simulink model "systemmodel"  (R2013b)
settings: Solver=ode45  StartTime=0.0  StopTime=10.0  RelTol=1e-3
values from neighbouring files (symbols this model uses):
  J_m1 = mean(J_1)    [identifier.m]
  J_m2 = mean(J_2)    [identifier.m]
  K_m1 = mean(k_1)    [identifier.m]
  K_m2 = mean(k_2)    [identifier.m]
undefined symbols (not defined in the file or in its folder): L_m1, L_m2
settings Model: Creator=torbal  LastModifiedBy=torbal

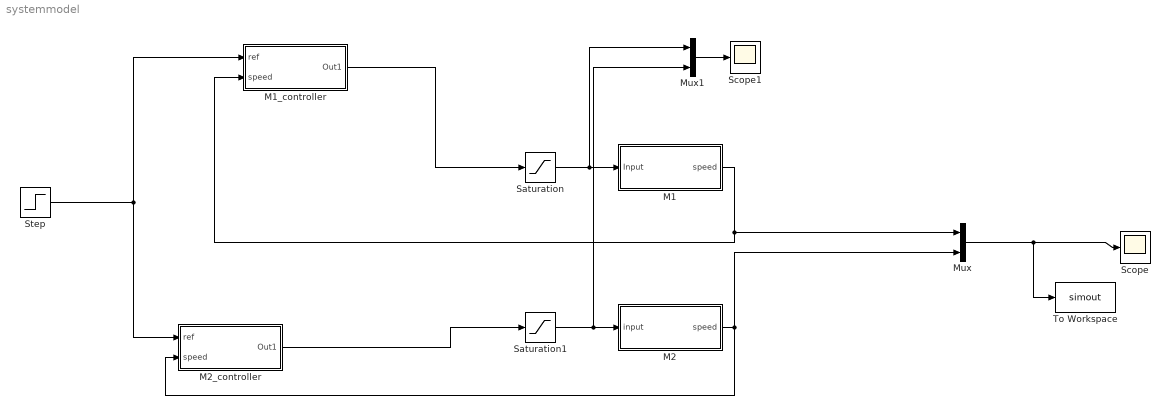
== system systemmodel ==
  M1 : Subsystem
  M1_controller : Subsystem
  M2 : Subsystem
  M2_controller : Subsystem
  Mux : Mux  Inputs=2
  Mux1 : Mux  Inputs=2
  Saturation : Saturate  UpperLimit=12  LowerLimit=-12
  Saturation1 : Saturate  UpperLimit=12  LowerLimit=-12
  Scope : Scope
      settings: TimeRange=10  YMin=0  YMax=60
  Scope1 : Scope
  Step : Step  After=50  SampleTime=0
  To Workspace : ToWorkspace  VariableName=simout  SampleTime=-1  SaveFormat=Timeseries
  wires:
  M2/1(speed) -> M2_controller/2(speed), Mux/2
  M1/1(speed) -> M1_controller/2(speed), Mux/1
  Mux/1 -> To Workspace/1, Scope/1
  M2_controller/1(Out1) -> Saturation1/1
  Saturation1/1 -> Mux1/2, M2/1(input)
  Saturation/1 -> Mux1/1, M1/1(Input)
  Mux1/1 -> Scope1/1
  Step/1 -> M1_controller/1("ref "), M2_controller/1("ref ")
  M1_controller/1(Out1) -> Saturation/1

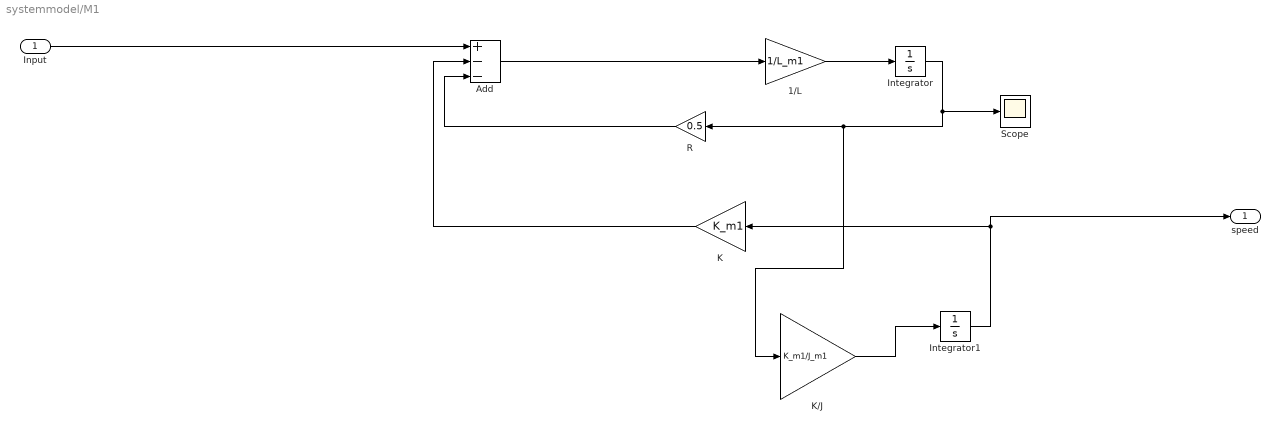
== system systemmodel/M1 ==
  Input : Inport
  1/L : Gain  Gain=1/L_m1
  Add : Sum  Inputs=+--
  Integrator : Integrator
  Integrator1 : Integrator
  K : Gain  Gain=K_m1
  K/J : Gain  Gain=K_m1/J_m1
  R : Gain  Gain=0.5
  Scope : Scope
      settings: SaveName=ScopeData2
  speed : Outport
  wires:
  1/L/1 -> Integrator/1
  Add/1 -> 1/L/1
  Input/1 -> Add/1
  K/J/1 -> Integrator1/1
  Integrator1/1 -> speed/1, K/1
  K/1 -> Add/2
  R/1 -> Add/3
  Integrator/1 -> K/J/1, R/1, Scope/1

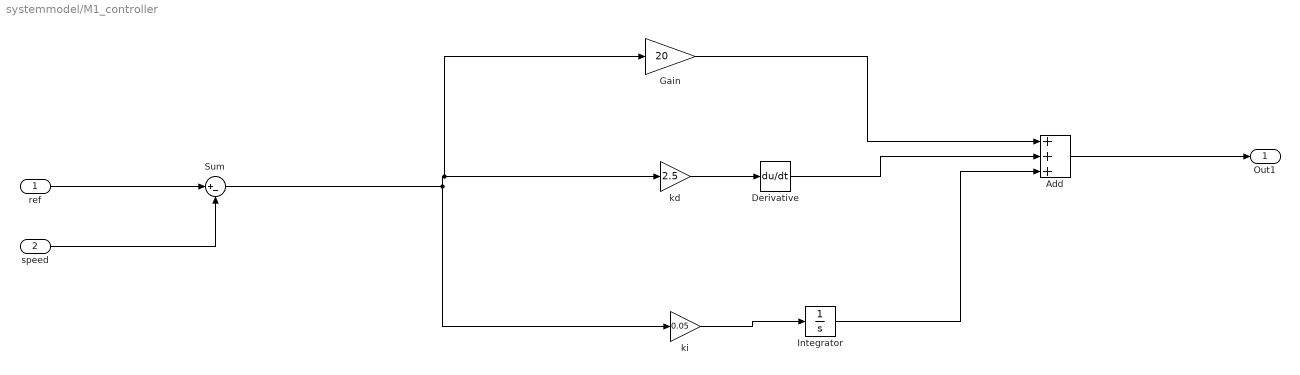
== system systemmodel/M1_controller ==
  "ref " : Inport
  speed : Inport  Port=2
  Add : Sum  Inputs=+++
  Derivative : Derivative
  Gain : Gain  Gain=20
  Integrator : Integrator
  Sum : Sum  Inputs=|+-
  "kd " : Gain  Gain=2.5
  ki : Gain  Gain=0.05
  Out1 : Outport
  wires:
  Gain/1 -> Add/1
  Add/1 -> Out1/1
  "ref "/1 -> Sum/1
  speed/1 -> Sum/2
  Sum/1 -> Gain/1, "kd "/1, ki/1
  "kd "/1 -> Derivative/1
  Derivative/1 -> Add/2
  ki/1 -> Integrator/1
  Integrator/1 -> Add/3

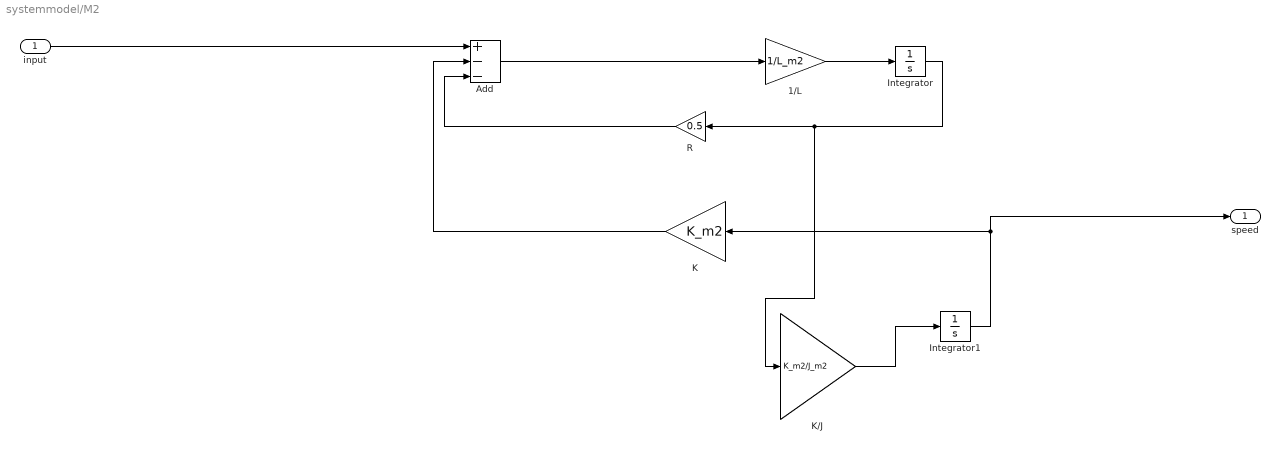
== system systemmodel/M2 ==
  input : Inport
  1/L : Gain  Gain=1/L_m2
  Add : Sum  Inputs=+--
  Integrator : Integrator
  Integrator1 : Integrator
  K : Gain  Gain=K_m2
  K/J : Gain  Gain=K_m2/J_m2
  R : Gain  Gain=0.5
  speed : Outport
  wires:
  1/L/1 -> Integrator/1
  Add/1 -> 1/L/1
  input/1 -> Add/1
  K/J/1 -> Integrator1/1
  Integrator1/1 -> speed/1, K/1
  K/1 -> Add/2
  Integrator/1 -> K/J/1, R/1
  R/1 -> Add/3

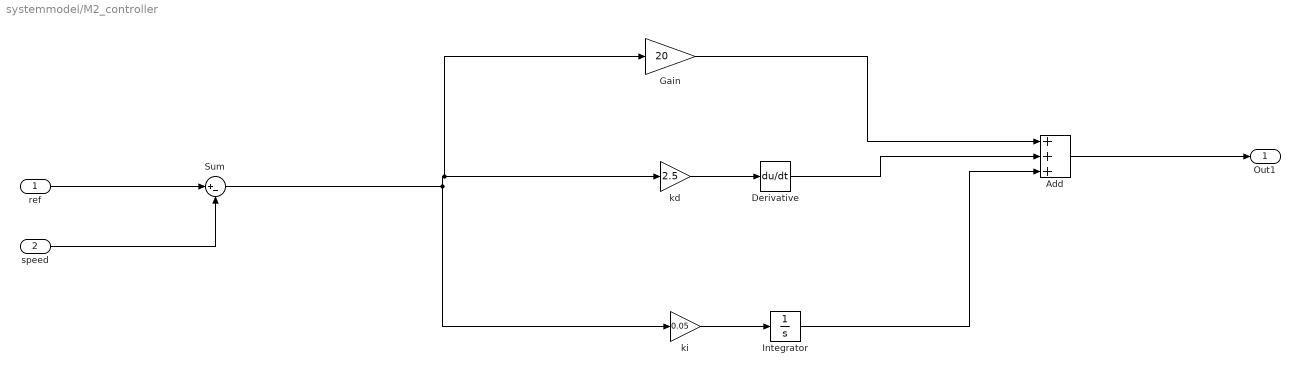
== system systemmodel/M2_controller ==
  "ref " : Inport
  speed : Inport  Port=2
  Add : Sum  Inputs=+++
  Derivative : Derivative
  Gain : Gain  Gain=20
  Integrator : Integrator
  Sum : Sum  Inputs=|+-
  "kd " : Gain  Gain=2.5
  ki : Gain  Gain=0.05
  Out1 : Outport
  wires:
  ki/1 -> Integrator/1
  Gain/1 -> Add/1
  Integrator/1 -> Add/3
  Add/1 -> Out1/1
  "ref "/1 -> Sum/1
  speed/1 -> Sum/2
  Sum/1 -> Gain/1, "kd "/1, ki/1
  "kd "/1 -> Derivative/1
  Derivative/1 -> Add/2
